simulink model "model_lab3_2"  (R2019b)
settings: Solver=VariableStepAuto  StartTime=0.0  StopTime=10.0  RelTol=1e-3
values from neighbouring files (symbols this model uses):
  A_c = [0 1;-I -N]    [zad_2.m]
  A_d = expm(h*A_c)    [zad_2.m]
  B_c = [0;1]    [zad_2.m]
  B_d = double(int(expm(t*A_c)*B_c,t,0,h))    [zad_2.m]
  C_c = [1 0; 0 1]    [zad_2.m]
  C_d = C_c    [zad_2.m]
  D_c = [0;0]    [zad_2.m]
  D_d = D_c    [zad_2.m]
  h = 1    [zad_2.m]
  WPC_c = WPC_d    (= 5)    [zad_2.m]
  WPC_d = 5    [zad_2.m]
settings Model: Creator=marci  LastModifiedBy=marci

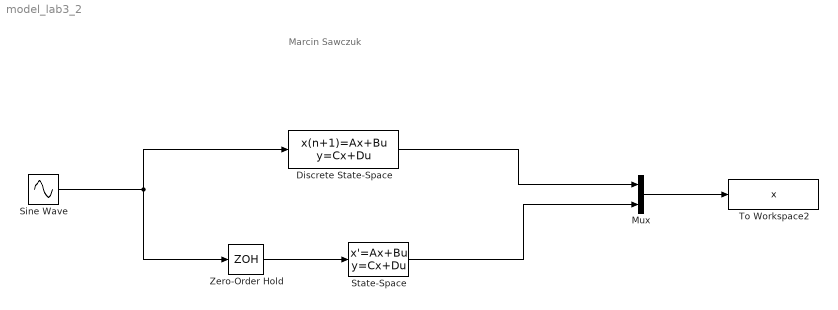
== system model_lab3_2 ==
  note: Marcin Sawczuk
  Discrete State-Space : DiscreteStateSpace  A=A_d  B=B_d  C=C_d  D=D_d  InitialCondition=WPC_d  SampleTime=h
  Mux : Mux  Inputs=2
  Sine Wave : Sin  SampleTime=0
  State-Space : StateSpace  A=A_c  B=B_c  C=C_c  D=D_c  InitialCondition=WPC_c
  To Workspace2 : ToWorkspace  VariableName=x  SampleTime=1e-2
  Zero-Order Hold : ZeroOrderHold  SampleTime=h
  wires:
  Discrete State-Space/1 -> Mux/1
  State-Space/1 -> Mux/2
  Sine Wave/1 -> Discrete State-Space/1, Zero-Order Hold/1
  Mux/1 -> To Workspace2/1
  Zero-Order Hold/1 -> State-Space/1
